simulink model "Tractor_KRAKER_etrailer_v2_2023a_backup050824"  (R2023a)
settings: Solver=VariableStepAuto  StartTime=0.0  StopTime=tmax  FixedStep=dt  RelTol=1e-3  EnableMultiTasking=on
PreLoadFcn:
  | init_vehicle
  | SIMSCAPE_BE_driveline_etrailer_parameters
StartFcn:
  | tic
StopFcn:
  | toc
  | sim_stop_function
  | Etrailer_Simscape_MBM_plotting
undefined symbols (not defined in the file): brake_input, chassis_length, end_val, energyCapacity, etrailer_ON, final_x, final_y, Floor, front_overhang, G, initialSOC, InputSwitch, L_0f, LD, mass_trailer, massload, MaxTrqOut, pose_t0, sp_t, Std_Regen_Trq, steer_input, steer_path, steer_ratio, steer_sens, throttle_input, tire_param_drive, tire_param_steer, tire_param_trailer, tire_width, v_0, Voc, Vx, Vx_input, wheelbase, X, Y, Z
libraries: sm_lib x367, nesl_utility x280, fl_lib x15, sdl_lib x2, robotalgslib x1, simulink_extras x1, batteryecm_lib x1, ee_lib x1, BatteryEstimators x1, CommercialVehicleLibrary2G x1
(part 2 of 12)

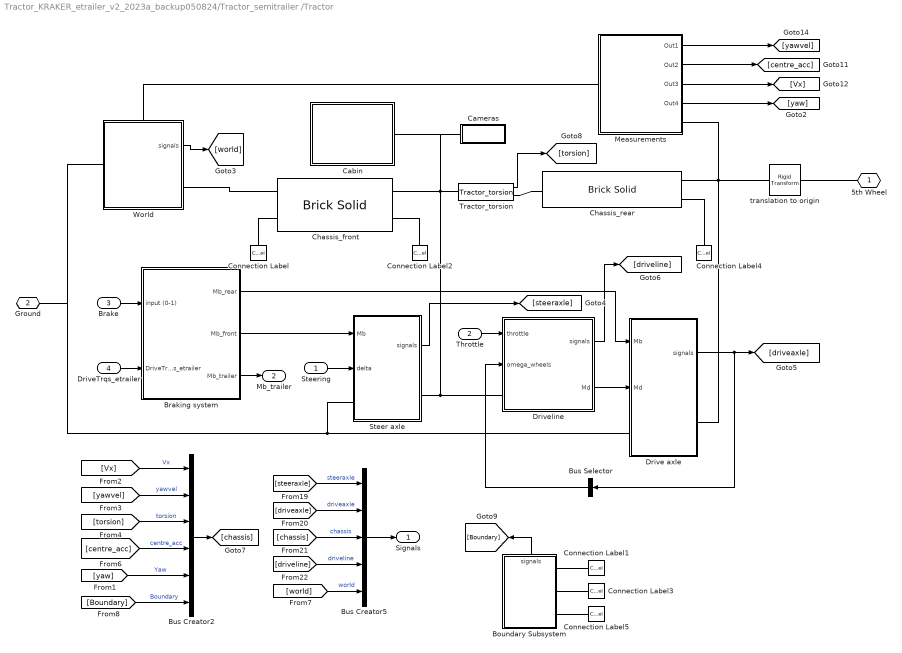
== system Tractor_KRAKER_etrailer_v2_2023a_backup050824/Tractor_semitrailer /Tractor ==
  Steering : Inport
  Throttle : Inport  Port=2
  Brake : Inport  Port=3
  DriveTrqs_etrailer : Inport  Port=4
  Boundary Subsystem : Subsystem
      settings: PortSchema="{\"entries\":[{\"content\":{\"sides\":[{\"content\":{},\"type\":\"ConnectorPlacement.EquallySpacedRectSide\",\"uuid\":\"f1bb1dfb-047a-4b1c-a7c6-7f55b7705282\"},{\"content\":{\"connectorIds\":[\"RConn1\",\"RConn2\",\"RConn3\"],\"side\":\"RIGHT\"},\"type\":\"ConnectorPlacement.EquallySpacedRectSide\",\"uuid\":\"a084a135-f208-49ed-a05d-7dd1e6403e76\"},{\"content\":{\"connectorIds\":[\"Out1\"],\"side\":\"TOP\"},\"type\":\"ConnectorPlacement.EquallySpacedRectSide\",\"uuid\":\"2d0c709c-7e4a-4964-89ae-6ca342da48b8\"},{\"content\":{\"side\":\"BOTTOM\"},\"type\":\"ConnectorPlacement.EquallySpacedRectSide\",\"uuid\":\"a753aab5-92ef-46fc-9973-c1109ebd78e0\"}]},\"type\":\"ConnectorPlacement.EquallySpacedConnector\",\"uuid\":\"ab4af6a2-1912-406b-b131-4cc7a9f5025c\"}],\"packageUris\":[\"http://schema.mathworks.com/mf0/Connector/R2020b\"],\"version\":\"1.0\"}"
      mask Display: disp('Boundary');
  Braking system : Subsystem  AncestorBlock=CommercialVehicleLibrary2G/Components/Braking system
  Bus Creator2 : BusCreator  Inputs=6
  Bus Creator5 : BusCreator  Inputs=5
  Bus Selector : BusSelector  OutputSignals=Omega1,Omega2  OutputAsBus=on
  Cabin : Subsystem  mask(cabin with coil/air suspension){xref=xref+1.10, zref=1.20}
      mask prompts: xref "global X-coordinate cabin tip point [m]"; zref "global Z-coordinate cabin tip point [m]"
      mask Display: disp('Cabin')
  Cameras : Subsystem
  Chassis_front : sm_lib/Body Elements/Brick Solid  GraphicAmbientColor=[0.15 0.15 0.15 1.0]  BasedOnType=Density  BrickDimensions=[l1 w1 h1]  BrickDimensionsUnits=m  CenterOfMass=[0 0 0]  CenterOfMassUnits=m  GraphicDiffuseColor=[0.4 0.4 0.4]  Density=1000  DensityUnits=kg/m^3  DoExposeReferenceFrame=on  GraphicEmissiveColor=[0.0 0.0 0.0 1.0]  ExportEntireGeometry=off  SerializedFrames=<Frames><Frame><Id>Frame1</Id><Value><Name>F1</Name><Origin><Source>ReferenceFrame</Source><FeatureName></FeatureName></Origin><PrimaryAxis><DefinedDirection>+Z</DefinedDirection><Source>ReferenceFrame</Source><SourceDirection>+Z</SourceDirection><FeatureName></FeatureName></PrimaryAxis><SecondaryAxis><DefinedDirection>+X</DefinedDirection><Source>ReferenceFrame</Source><SourceDirection>+X</SourceDirection><FeatureName></FeatureName></SecondaryAxis></Value></Frame><Frame><Id>Frame2</Id><Value><Name>Front</Name><Origin><Source>GeometricFeature</Source><FeatureName>+x surface</FeatureName></Origin><PrimaryAxis><DefinedDirection>+Z</DefinedDirection><Source>ReferenceFrame</Source><SourceDirection>+Z</SourceDirection><FeatureName></FeatureName></PrimaryAxis><SecondaryAxis><DefinedDirection>+X</DefinedDirection><Source>ReferenceFrame</Source><SourceDirection>+X</SourceDirection><FeatureName></FeatureName></SecondaryAxis></Value></Frame><Frame><Id>Frame3</Id><Value><Name>Center</Name><Origin><Source>GeometricFeature</Source><FeatureName>-x surface</FeatureName></Origin><PrimaryAxis><DefinedDirection>+Z</DefinedDirection><Source>ReferenceFrame</Source><SourceDirection>+Z</SourceDirection><FeatureName></FeatureName></PrimaryAxis><SecondaryAxis><DefinedDirection>+X</DefinedDirection><Source>ReferenceFrame</Source><SourceDirection>+X</SourceDirection><FeatureName></FeatureName></SecondaryAxis></Value></Frame></Frames>  MarkerShape=Sphere  MarkerSize=10  GraphicType=FromGeometry  InertiaType=Custom  Mass=front_mass  MassUnits=kg  MomentsOfInertia=[front_Ixx front_Iyy front_Izz]  MomentsOfInertiaUnits=kg*m^2  GraphicOpacity=1  ProductsOfInertia=[0 0 0]  ProductsOfInertiaUnits=kg*m^2  GraphicShininess=75  GraphicSpecularColor=[0.5 0.5 0.5 1.0]  GraphicVisPropType=SimpleVisualProperties
  Chassis_rear : sm_lib/Body Elements/Brick Solid  GraphicAmbientColor=[0.15 0.15 0.15 1.0]  BasedOnType=Density  BrickDimensions=[l2 w2 h2]  BrickDimensionsUnits=m  CenterOfMass=[0 0 0]  CenterOfMassUnits=m  GraphicDiffuseColor=[0.9 0.9 0.9]  Density=1000  DensityUnits=kg/m^3  DoExposeReferenceFrame=on  GraphicEmissiveColor=[0.0 0.0 0.0 1.0]  ExportEntireGeometry=off  SerializedFrames=<Frames><Frame><Id>Frame1</Id><Value><Name>F1</Name><Origin><Source>ReferenceFrame</Source><FeatureName></FeatureName></Origin><PrimaryAxis><DefinedDirection>+Z</DefinedDirection><Source>ReferenceFrame</Source><SourceDirection>+Z</SourceDirection><FeatureName></FeatureName></PrimaryAxis><SecondaryAxis><DefinedDirection>+X</DefinedDirection><Source>ReferenceFrame</Source><SourceDirection>+X</SourceDirection><FeatureName></FeatureName></SecondaryAxis></Value></Frame><Frame><Id>Frame2</Id><Value><Name>Rear</Name><Origin><Source>GeometricFeature</Source><FeatureName>-x surface</FeatureName></Origin><PrimaryAxis><DefinedDirection>+Z</DefinedDirection><Source>ReferenceFrame</Source><SourceDirection>+Z</SourceDirection><FeatureName></FeatureName></PrimaryAxis><SecondaryAxis><DefinedDirection>+X</DefinedDirection><Source>ReferenceFrame</Source><SourceDirection>+X</SourceDirection><FeatureName></FeatureName></SecondaryAxis></Value></Frame></Frames>  MarkerShape=Sphere  MarkerSize=10  GraphicType=FromGeometry  InertiaType=Custom  Mass=rear_mass  MassUnits=kg  MomentsOfInertia=[rear_Ixx rear_Iyy rear_Izz]  MomentsOfInertiaUnits=kg*m^2  GraphicOpacity=0.8  ProductsOfInertia=[0 0 0]  ProductsOfInertiaUnits=kg*m^2  GraphicShininess=75  GraphicSpecularColor=[0.5 0.5 0.5 1.0]  GraphicVisPropType=SimpleVisualProperties
  Connection Label : ConnectionLabel  Label=Center
  Connection Label1 : ConnectionLabel  Label=Center
  Connection Label2 : ConnectionLabel  Label=Front
  Connection Label3 : ConnectionLabel  Label=Front
  Connection Label4 : ConnectionLabel  Label=Rear
  Connection Label5 : ConnectionLabel  Label=Rear
  Drive axle : Subsystem  mask(Driven axle with double tyres){xpos=xref+xrear, tire_param=tire_param_drive, Vx=Vx, Fzstat=Fzstat2}
      mask prompts: xpos "global X-coordinate wheelcentre [m]"; tire_param "tire parameters (structure)"; Vx "initial velocity Vx [m/s]"; Fzstat "initial vertical axle load [N]"
      mask init:
      | Rtyre     = 0.548;
      | Cztyre    = 1.13e+006;
      | tyre_mass = tire_param.INERTIA.MASS;
      | 
      | zpos = Rtyre - 0.25*Fzstat/Cztyre;
      | 
      | tw  =2.15;    % [m], track_width outer tyres
      | ywhl=0.35;   % [m], distance between double tyres
      | yd  =1.00;    % [m], Y-distance bewteen dampers
      | ys  =0.75;    % [m], Y-distance bewteen springs
      | zrc =0.30;   % [m], height of roll centre wrt axle centre 
      | 
      | % damping/stiffness
      | Kspring = 320000;    % [N/m], spring stiffness  (two per axle!)
      | Bdamper =  15000;    % [Ns/m], damper constant  (two per axle!)
      | Kroll   = 500000;    % [Nm/rad] roll stiffness 
      | 
      | % mass/inertia
      | axle_mass =1000;     % [kg] (excl. wheels/tyres!)
      | axle_Ixx  = 380;     % [kgm2]
      | axle_Iyy  =  10;     % [kgm2]
      | axle_Izz  = 380;     % [kgm2]
      |    
      | %rim
      | rim_mass= 50;        % [kg]
      | rim_Ixx =  3;        % [kgm2]
      | rim_Iyy =  5;        % [kgm2] (including rotational inertia brake disk)
      | 
      | %WHeel mass 
      | wheelbody_mass = rim_mass + tire_param.INERTIA.MASS;
      | wheelbody_Ixx  = rim_Ixx  + tire_param.INERTIA.IXX;
      | wheelbody_Iyy  = rim_Iyy  + tire_param.INERTIA.IYY;
      | Imat = [wheelbody_Ixx 0 0; 0 wheelbody_Iyy 0; 0 0 wheelbody_Ixx];
      | sideR=-1;
      | sideL=1;
      | 
      | ld = 0.3;            % loaded spring/damper length
      | ls = ld + 0.5*(Fzstat - 9.81*(axle_mass + 4*tyre_mass + 4*rim_mass))/Kspring;  % spring unloaded length
      settings: LibrarySourceBlock=CommercialVehicleLibrary2G/Assemblies/Drive axle
  Driveline : Subsystem  mask(Engine+gearbox){xref=xref-0.162, zref=0.58, param=DAF XEC + TC-Tronic (355 kW/2100 Nm)}
      mask prompts: xref "global X-coordinate engine ref. point [m]"; zref "global Z-coordinate engine ref. point [m]"; param "parameters"
      mask init:
      | % engine/gearbox: DAF XE355C / ZF 16S221
      | eng_power         = 355000;  % 355 kW
      | max_engine_torque = 2100;    % [Nm]
      | max_revs_rpm      = 1900;    % [rpm]
      | first_gear_ratio  = 16.41;   % [-]
      | final_drive_ratio =  3.07;   % [-]
      |  
      | % engine + gearbox mass (XEC +TC-tronic, DAF 51051/03-042 R. Liebrechts)
      | driveline_mass= 1800;       %[kg]
      | Ixx =  100;       %[kgm2]
      | Iyy =  900;       %[kgm2]
      | Izz =  900;       %[kgm2]
      | yrot=   0;        %[rad] rotation about Y-axis of inertial frame
      | xcg =  -0.25;     %[m], X-coordinate CG wrt rear engine mount ref. point
      | zcg =   0.30;     %[m], Z-coordinate CG wrt rear engine mount ref. point
      |  
      | omega_max=2*pi*max_revs_rpm/60;
      mask TypeOptions param: DAF XEC + TC-Tronic (355 kW/2100 Nm)
  Measurements : Subsystem
  Steer axle : Subsystem  mask(Axle with single tyres and steering system){xpos=xref, tire_param=tire_param_steer, Vx=Vx, Fzstat=Fzstat1}
      mask prompts: xpos "global X-coordinate wheelcentre [m]"; tire_param "tire parameters (structure)"; Vx "initial velocity Vx [m/s]"; Fzstat "initial vertical axle load [N]"
      mask init:
      | Rtyre    = 0.548;
      | Cztyre   = 1.19e+006;
      | tyre_mass= tire_param.INERTIA.MASS;
      | 
      | zpos=Rtyre - 0.5*Fzstat/Cztyre;
      | 
      | steerratio = 20; %[-], ratio steering wheel - front wheels
      |  
      | % dimensions
      | tw =2.0; 	% [m], track_width
      | zrc=0;    	% [m], height of roll centre wrt axle centerline   
      | yd =1.0; 	% [m], Y-distance bewteen dampers 
      | ys =0.85; 	% [m], Y-distance bewteen springs
      | 
      | % stiffness/damping
      | Kspring = 300000;  	% [N/m], spring stiffness (two per axle!)
      | Bdamper =  15000;  	% [Ns/m] damper constant  (two per axle!)
      | Kroll   = 200000;  	% [Nm/rad], roll stiffness 
      |    
      | % mass/inertia   
      | axle_mass = 475;    % [kg] (excl. wheels/tyres!)
      | axle_Ixx  = 200;	% [kgm2]
      | axle_Iyy  = 5;      % [kgm2]
      | axle_Izz  = 200;	% [kgm2]
      |    
      | %rim mass
      | rim_mass= 50; 	% [kg]
      | rim_Ixx =  3; 	% [kgm2]
      | rim_Iyy =  5; 	% [kgm2] (including rotational inertia brake disk)
      | 
      | %WHeel mass 
      | wheelbody_mass = rim_mass + tire_param.INERTIA.MASS;
      | wheelbody_Ixx  = rim_Ixx  + tire_param.INERTIA.IXX;
      | wheelbody_Iyy  = rim_Iyy  + tire_param.INERTIA.IYY;
      | Imat = [wheelbody_Ixx 0 0; 0 wheelbody_Iyy 0; 0 0 wheelbody_Ixx];
      | sideR=-1;
      | sideL=1;
      | 
      | ld = 0.3;       % loaded spring/damper length
      | ls = ld + 0.5*(Fzstat - 9.81*(axle_mass + 2*tyre_mass + 2*rim_mass))/Kspring;  % spring unloaded length
      settings: LibrarySourceBlock=CommercialVehicleLibrary2G/Assemblies/Steer axle
  Tractor_torsion : CommercialVehicleLibrary2G/Components/Tractor_torsion
      mask Display: disp('Torsion');
  World : Subsystem
      settings: LibrarySourceBlock=CommercialVehicleLibrary2G/Utilities/World  PortSchema="{\"entries\":[{\"content\":{\"sides\":[{\"content\":{\"connectorIds\":[\"LConn1\"]},\"type\":\"ConnectorPlacement.EquallySpacedRectSide\",\"uuid\":\"a76c8e8f-6db3-49af-b69e-3287a57a87d6\"},{\"content\":{\"connectorIds\":[\"Out1\",\"RConn1\"],\"side\":\"RIGHT\"},\"type\":\"ConnectorPlacement.EquallySpacedRectSide\",\"uuid\":\"762bfe49-08bc-424a-9ad2-f8d2880b424d\"},{\"content\":{\"connectorIds\":[\"LConn2\"],\"side\":\"TOP\"},\"type\":\"ConnectorPlacement.EquallySpacedRectSide\",\"uuid\":\"ab579a77-7604-4f94-9589-5926789d5e9b\"}]},\"type\":\"ConnectorPlacement.EquallySpacedConnector\",\"uuid\":\"89dbc719-7b2e-4b66-8c99-9a61a858c760\"}],\"packageUris\":[\"http://schema.mathworks.com/mf0/Connector/R2020b\"],\"version\":\"1.0\"}"
  translation to origin : sm_lib/Frames and Transforms/Rigid Transform  TranslationMethod=Cartesian  TranslationStandardOffset=0  TranslationStandardOffsetUnits=m  TranslationStandardAxis=+Z  TranslationCartesianOffset=[-xcg_rear 0 -0.9]  TranslationCartesianOffsetUnits=m  TranslationROffset=0  TranslationROffsetUnits=m  TranslationZOffset=0  TranslationZOffsetUnits=m  TranslationThetaOffset=0  TranslationThetaOffsetUnits=deg  RotationMethod=None  RotationAngleUnits=deg  RotationStandardAxis=+Z  RotationAngle=0.0  RotationArbitraryAxis=[0 0 1]  FollAlignAxisA=+Z  BaseAlignAxisA=+X  FollAlignAxisB=+Y  BaseAlignAxisB=+Y  RotationSequenceAxes=FollowerAxes  RotationSequence=XYX  RotationSequenceAngles=[0 0 0]  RotationSequenceAnglesUnits=deg  RotationMatrix=[1 0 0; 0 1 0; 0 0 1]  Quaternion=[1 0 0 0]
  5th Wheel : PMIOPort  Tag=PMCPort  Side=Right
  Ground : PMIOPort  Port=2  Side=Right
  Signals : Outport
  Mb_trailer : Outport  Port=2
  wires:
  [yawvel] -> Bus Creator2/2  "yawvel"
  Bus Creator2/1 -> [chassis]
  [centre_acc] -> Bus Creator2/4  "centre_acc"
  [torsion] -> Bus Creator2/3  "torsion"
  [Vx] -> Bus Creator2/1  "Vx"
  Tractor_torsion/1 -> [torsion]
  Measurements/3(Out3) -> [Vx]
  Measurements/1(Out1) -> [yawvel]
  Measurements/2(Out2) -> [centre_acc]
  Steer axle/1(signals) -> [steeraxle]
  Drive axle/1(signals) -> Bus Selector/1, [driveaxle]
  Braking system/3(Mb_trailer) -> Mb_trailer/1
  Brake/1 -> Braking system/1(input (0-1))
  Throttle/1 -> Driveline/1(throttle)
  Bus Selector/1 -> Driveline/2(omega_wheels)
  Driveline/2(Md) -> Drive axle/2(Md)
  Steering/1 -> Steer axle/2(delta)
  Driveline/1(signals) -> [driveline]
  [steeraxle] -> Bus Creator5/1  "steeraxle"
  [driveaxle] -> Bus Creator5/2  "driveaxle"
  [chassis] -> Bus Creator5/3  "chassis"
  [driveline] -> Bus Creator5/4  "driveline"
  Bus Creator5/1 -> Signals/1
  Braking system/1(Mb_rear) -> Drive axle/1(Mb)
  Braking system/2(Mb_front) -> Steer axle/1(Mb)
  Measurements/4(Out4) -> [yaw]
  [yaw] -> Bus Creator2/5  "Yaw"
  World/1(signals) -> [world]
  [world] -> Bus Creator5/5  "world"
  Boundary Subsystem/1(signals) -> [Boundary]
  [Boundary] -> Bus Creator2/6  "Boundary"
  DriveTrqs_etrailer/1 -> Braking system/2(DriveTrqs_etrailer)
  connections:
  5th Wheel/RConn1 -- translation to origin/RConn1
  World/RConn1 -- Chassis_front/RConn1
  Chassis_rear/RConn1 -- Tractor_torsion/RConn1
  translation to origin/LConn1 -- Drive axle/RConn1 -- Chassis_rear/LConn1 -- Measurements/RConn1
  World/LConn2 -- Measurements/LConn1
  Steer axle/RConn1 -- Driveline/LConn1 -- Chassis_front/LConn1 -- Cabin/RConn1 -- Cameras/LConn1 -- Tractor_torsion/LConn1
  Drive axle/LConn1 -- Steer axle/LConn1 -- World/LConn1 -- Ground/RConn1
  Chassis_front/RConn2 -- Connection Label/LConn1
  Connection Label1/LConn1 -- Boundary Subsystem/RConn1
  Chassis_front/LConn2 -- Connection Label2/LConn1
  Connection Label3/LConn1 -- Boundary Subsystem/RConn2
  Chassis_rear/LConn2 -- Connection Label4/LConn1
  Connection Label5/LConn1 -- Boundary Subsystem/RConn3

== system Tractor_KRAKER_etrailer_v2_2023a_backup050824/Tractor_semitrailer /Driver/Control ==
  path : Inport
  truck_x : Inport  Port=2
  truck_y : Inport  Port=3
  truck_yaw : Inport  Port=4
  Mux : Mux  Inputs=3
  Pure persuit controller : Subsystem
  Radians to Degrees1 : simulink_extras/Transformations/Radians to Degrees  Commented=on
  Rate Limiter1 : RateLimiter  Commented=on  RisingSlewLimit=0.9  FallingSlewLimit=-0.9  SampleTimeMode=inherited
  Saturation 45 to -45 deg : Saturate  UpperLimit=0.78539816  LowerLimit=-0.78539816
  Simulation end module : Subsystem  Commented=on
  Steering ratio and sens : Gain  Gain=steer_ratio*steer_sens
  delta in rad : Outport
  wires:
  truck_yaw/1 -> Mux/3
  path/1 -> Pure persuit controller/2(Waypoints)
  Pure persuit controller/1(Delta) -> Saturation 45 to -45 deg/1  "delta_C"
  truck_x/1 -> Simulation end module/1(x), Mux/1
  truck_y/1 -> Simulation end module/2(y), Mux/2
  Mux/1 -> Pure persuit controller/1(Pose)
  Steering ratio and sens/1 -> delta in rad/1
  Saturation 45 to -45 deg/1 -> Steering ratio and sens/1

== system Tractor_KRAKER_etrailer_v2_2023a_backup050824/Tractor_semitrailer /Driver/CruiseControl ==
  Vx,ref : Inport
  Vx,actual : Inport  Port=2
  Add : Sum  Inputs=+-
  Add1 : Sum
  Gain : Gain  Gain=5
  Gain1 : Gain  Gain=5
  Integrator : Integrator  InitialCondition=0.0  LimitOutput=on  UpperSaturationLimit=0.1  LowerSaturationLimit=-0.1
  Lookup Table : Lookup  InputValues="[-10  2  10 30]"  Table=[0.04 0.04 1 1]  SaturateOnIntegerOverflow=off
  Product : Product  RndMeth=Zero
  Product1 : Product  RndMeth=Zero
  Scope : Scope  NumInputPorts=2
  To Workspace : ToWorkspace  VariableName=p_velocity_reference  SampleTime=sp_t
  To Workspace1 : ToWorkspace  VariableName=p_velocity_actual  SampleTime=sp_t
  Transfer Fcn : TransferFcn  Denominator=[0.16 1]
  throttle : Outport  VectorParamsAs1DForOutWhenUnconnected=off
  wires:
  Transfer Fcn/1 -> Lookup Table/1
  Lookup Table/1 -> Product/2, Product1/2
  Product1/1 -> Gain1/1
  Product/1 -> Gain/1
  Add/1 -> Product1/1, Product/1
  Add1/1 -> throttle/1
  Gain/1 -> Add1/1
  Integrator/1 -> Add1/2
  Gain1/1 -> Integrator/1
  Vx,ref/1 -> To Workspace/1, Scope/1, Add/1
  Vx,actual/1 -> Transfer Fcn/1, To Workspace1/1, Scope/2, Add/2

== system Tractor_KRAKER_etrailer_v2_2023a_backup050824/Tractor_semitrailer /Driver/Subsystem ==
  Constant : Constant  Value=InputSwitch
  DriveCycle Speed Input : FromWorkspace  VariableName=DrCycles.FTP
  From Workspace : FromWorkspace  VariableName=DrCycles.C505
  From Workspace1 : FromWorkspace  VariableName=DrCycles.UDDS
  From Workspace2 : FromWorkspace  VariableName=DrCycles.HWFET
  From Workspace3 : FromWorkspace  VariableName=DrCycles.US06
  From Workspace4 : FromWorkspace  VariableName=DrCycles.US06City
  From Workspace5 : FromWorkspace  VariableName=DrCycles.US06Hwy
  Multiport Switch : MultiPortSwitch  Inputs=8  SaturateOnIntegerOverflow=off  InputSameDT=off
  Saturation : Saturate  UpperLimit=90  LowerLimit=0
  SineWave DriveCycle Input : Sin  Amplitude=150  Bias=50  Frequency=0.1  SampleTime=0
  mph2mps{,1..6} (7 alike) : Gain  Gain=0.44704
  DriveCycleInput : Outport
  wires:
  SineWave DriveCycle Input/1 -> Saturation/1
  DriveCycle Speed Input/1 -> mph2mps/1
  mph2mps/1 -> Multiport Switch/2
  Constant/1 -> Multiport Switch/1
  Multiport Switch/1 -> DriveCycleInput/1
  mph2mps1/1 -> Multiport Switch/3
  From Workspace/1 -> mph2mps1/1
  mph2mps2/1 -> Multiport Switch/4
  From Workspace1/1 -> mph2mps2/1
  mph2mps3/1 -> Multiport Switch/5
  mph2mps4/1 -> Multiport Switch/6
  mph2mps5/1 -> Multiport Switch/7
  mph2mps6/1 -> Multiport Switch/8
  From Workspace2/1 -> mph2mps3/1
  From Workspace3/1 -> mph2mps4/1
  From Workspace4/1 -> mph2mps5/1
  From Workspace5/1 -> mph2mps6/1
  Saturation/1 -> Multiport Switch/9

== system Tractor_KRAKER_etrailer_v2_2023a_backup050824/Tractor_semitrailer /Kraker etrailer/5th Wheel Joint ==
  note: 2 Joint setup
  note: 1 joint setup
  note: Signals for forces on kingpin
  note: in X-Z-Y
  note: in X-Z-Y
  note: in X-Y-Z
  note: in X-Y-Z
  note: in Z-Y-X
  note: in Z-Y-X
  5th wheel joint : sm_lib/Joints/Revolute Joint  Commented=on  JointMode=Normal  SenseConstraintForce=on  SenseConstraintForceX=off  SenseConstraintForceY=off  SenseConstraintForceZ=off  SenseConstraintTorque=off  SenseConstraintTorqueX=off  SenseConstraintTorqueY=off  SenseConstraintTorqueZ=off  SenseTotalForce=on  SenseTotalForceX=off  SenseTotalForceY=off  SenseTotalForceZ=off  SenseTotalTorque=off  SenseTotalTorqueX=off  SenseTotalTorqueY=off  SenseTotalTorqueZ=off  CompositeWrenchDir=BaseOnFollower  CompositeWrenchFrame=BaseFrame  EquilibriumPosition=0  EquilibriumPositionUnits=deg  SpringStiffness=0  SpringStiffnessUnits=N*m/deg  DampingCoefficient=0  DampingCoefficientUnits=N*m/(deg/s)  TorqueActuationMode=NoTorque  MotionActuationMode=ComputedMotion  SensePosition=off  SenseVelocity=off  SenseAcceleration=off  SenseTorqueForce=off  SenseLowerLimitTorqueForce=off  SenseUpperLimitTorqueForce=off  LowerLimitSpecify=off  LowerLimitBound=-90  LowerLimitBoundUnits=deg  LowerLimitStiffness=1e4  LowerLimitStiffnessUnits=N*m/deg  LowerLimitDamping=10  LowerLimitDampingUnits=N*m/(deg/s)  LowerLimitTransitionRegionWidth=0.1  LowerLimitTransitionRegionWidthUnits=deg  UpperLimitSpecify=off  UpperLimitBound=90  UpperLimitBoundUnits=deg  UpperLimitStiffness=1e4  UpperLimitStiffnessUnits=N*m/deg  UpperLimitDamping=10  UpperLimitDampingUnits=N*m/(deg/s)  UpperLimitTransitionRegionWidth=0.1  UpperLimitTransitionRegionWidthUnits=deg  PositionTargetSpecify=on  PositionTargetPriority=High  PositionTargetValue=-psi_semitrailer  PositionTargetValueUnits=rad  VelocityTargetSpecify=off  VelocityTargetPriority=High  VelocityTargetValue=0  VelocityTargetValueUnits=deg/s
  5th wheel joint - axis : sm_lib/Joints/Revolute Joint  Commented=on  JointMode=Normal  SenseConstraintForce=on  SenseConstraintForceX=off  SenseConstraintForceY=off  SenseConstraintForceZ=off  SenseConstraintTorque=off  SenseConstraintTorqueX=off  SenseConstraintTorqueY=off  SenseConstraintTorqueZ=off  SenseTotalForce=on  SenseTotalForceX=off  SenseTotalForceY=off  SenseTotalForceZ=off  SenseTotalTorque=off  SenseTotalTorqueX=off  SenseTotalTorqueY=off  SenseTotalTorqueZ=off  CompositeWrenchDir=FollowerOnBase  CompositeWrenchFrame=BaseFrame  EquilibriumPosition=0  EquilibriumPositionUnits=deg  SpringStiffness=0  SpringStiffnessUnits=N*m/deg  DampingCoefficient=0  DampingCoefficientUnits=N*m/(deg/s)  TorqueActuationMode=NoTorque  MotionActuationMode=ComputedMotion  SensePosition=off  SenseVelocity=off  SenseAcceleration=off  SenseTorqueForce=off  SenseLowerLimitTorqueForce=off  SenseUpperLimitTorqueForce=off  LowerLimitSpecify=off  LowerLimitBound=-90  LowerLimitBoundUnits=deg  LowerLimitStiffness=1e4  LowerLimitStiffnessUnits=N*m/deg  LowerLimitDamping=10  LowerLimitDampingUnits=N*m/(deg/s)  LowerLimitTransitionRegionWidth=0.1  LowerLimitTransitionRegionWidthUnits=deg  UpperLimitSpecify=off  UpperLimitBound=90  UpperLimitBoundUnits=deg  UpperLimitStiffness=1e4  UpperLimitStiffnessUnits=N*m/deg  UpperLimitDamping=10  UpperLimitDampingUnits=N*m/(deg/s)  UpperLimitTransitionRegionWidth=0.1  UpperLimitTransitionRegionWidthUnits=deg  PositionTargetSpecify=off  PositionTargetPriority=High  PositionTargetValue=0  PositionTargetValueUnits=deg  VelocityTargetSpecify=off  VelocityTargetPriority=High  VelocityTargetValue=0  VelocityTargetValueUnits=deg/s
  Align : sm_lib/Frames and Transforms/Rigid Transform  TranslationMethod=None  TranslationStandardOffset=0  TranslationStandardOffsetUnits=m  TranslationStandardAxis=+Z  TranslationCartesianOffset=[0 0 0]  TranslationCartesianOffsetUnits=m  TranslationROffset=0  TranslationROffsetUnits=m  TranslationZOffset=0  TranslationZOffsetUnits=m  TranslationThetaOffset=0  TranslationThetaOffsetUnits=deg  RotationMethod=AlignedAxes  RotationAngleUnits=deg  RotationStandardAxis=+Z  RotationAngle=0.0  RotationArbitraryAxis=[0 0 1]  FollAlignAxisA=+X  BaseAlignAxisA=+Z  FollAlignAxisB=+Y  BaseAlignAxisB=+Y  RotationSequenceAxes=FollowerAxes  RotationSequence=XYX  RotationSequenceAngles=[0 0 0]  RotationSequenceAnglesUnits=deg  RotationMatrix=[1 0 0; 0 1 0; 0 0 1]  Quaternion=[1 0 0 0]
  Align_5th wheel : sm_lib/Frames and Transforms/Rigid Transform  Commented=on  TranslationMethod=None  TranslationStandardOffset=0  TranslationStandardOffsetUnits=m  TranslationStandardAxis=+Z  TranslationCartesianOffset=[0 0 0]  TranslationCartesianOffsetUnits=m  TranslationROffset=0  TranslationROffsetUnits=m  TranslationZOffset=0  TranslationZOffsetUnits=m  TranslationThetaOffset=0  TranslationThetaOffsetUnits=deg  RotationMethod=AlignedAxes  RotationAngleUnits=deg  RotationStandardAxis=+Z  RotationAngle=0.0  RotationArbitraryAxis=[0 0 1]  FollAlignAxisA=+Z  BaseAlignAxisA=+Y  FollAlignAxisB=+X  BaseAlignAxisB=+X  RotationSequenceAxes=FollowerAxes  RotationSequence=XYX  RotationSequenceAngles=[0 0 0]  RotationSequenceAnglesUnits=deg  RotationMatrix=[1 0 0; 0 1 0; 0 0 1]  Quaternion=[1 0 0 0]
  Bus Creator : BusCreator  Inputs=3
  Bus Creator1 : BusCreator  Inputs=5
  Goto1 : Goto  Commented=on  GotoTag=Ft_Joint1
  Goto2 : Goto  Commented=on  GotoTag=Fc_Joint1
  Goto3 : Goto  Commented=on  GotoTag=Ft_Joint2
  Goto4 : Goto  Commented=on  GotoTag=Fc_Joint2
  PS-Simulink Converter : nesl_utility/PS-Simulink Converter  PhysicalDomain=network_engine_domain  SubClassName=ps_output  LeftPortType=input  RightPortType=output  PseudoPeriodic=off  Frequencies=[]  VectorFormat=1-D array  Unit=inherit  AffineConversion=off
  PS-Simulink Converter1 : nesl_utility/PS-Simulink Converter  PhysicalDomain=network_engine_domain  SubClassName=ps_output  LeftPortType=input  RightPortType=output  PseudoPeriodic=off  Frequencies=[]  VectorFormat=1-D array  Unit=inherit  AffineConversion=off
  PS-Simulink Converter10 : nesl_utility/PS-Simulink Converter  PhysicalDomain=network_engine_domain  SubClassName=ps_output  LeftPortType=input  RightPortType=output  PseudoPeriodic=off  Frequencies=[]  VectorFormat=1-D array  Unit=deg  AffineConversion=off
  PS-Simulink Converter2 : nesl_utility/PS-Simulink Converter  PhysicalDomain=network_engine_domain  SubClassName=ps_output  LeftPortType=input  RightPortType=output  PseudoPeriodic=off  Frequencies=[]  VectorFormat=1-D array  Unit=inherit  AffineConversion=off
  PS-Simulink Converter{3..6} (4 alike) : nesl_utility/PS-Simulink Converter  Commented=on  PhysicalDomain=network_engine_domain  SubClassName=ps_output  LeftPortType=input  RightPortType=output  PseudoPeriodic=off  Frequencies=[]  VectorFormat=1-D array  Unit=N  AffineConversion=off
  PS-Simulink Converter8 : nesl_utility/PS-Simulink Converter  PhysicalDomain=network_engine_domain  SubClassName=ps_output  LeftPortType=input  RightPortType=output  PseudoPeriodic=off  Frequencies=[]  VectorFormat=1-D array  Unit=N  AffineConversion=off
  PS-Simulink Converter9 : nesl_utility/PS-Simulink Converter  PhysicalDomain=network_engine_domain  SubClassName=ps_output  LeftPortType=input  RightPortType=output  PseudoPeriodic=off  Frequencies=[]  VectorFormat=1-D array  Unit=N  AffineConversion=off
  Realign : sm_lib/Frames and Transforms/Rigid Transform  TranslationMethod=None  TranslationStandardOffset=0  TranslationStandardOffsetUnits=m  TranslationStandardAxis=+Z  TranslationCartesianOffset=[0 0 0]  TranslationCartesianOffsetUnits=m  TranslationROffset=0  TranslationROffsetUnits=m  TranslationZOffset=0  TranslationZOffsetUnits=m  TranslationThetaOffset=0  TranslationThetaOffsetUnits=deg  RotationMethod=AlignedAxes  RotationAngleUnits=deg  RotationStandardAxis=+Z  RotationAngle=0.0  RotationArbitraryAxis=[0 0 1]  FollAlignAxisA=+Z  BaseAlignAxisA=+X  FollAlignAxisB=+Y  BaseAlignAxisB=+Y  RotationSequenceAxes=FollowerAxes  RotationSequence=XYX  RotationSequenceAngles=[0 0 0]  RotationSequenceAnglesUnits=deg  RotationMatrix=[1 0 0; 0 1 0; 0 0 1]  Quaternion=[1 0 0 0]
  Realign_5th wheel : sm_lib/Frames and Transforms/Rigid Transform  Commented=on  TranslationMethod=None  TranslationStandardOffset=0  TranslationStandardOffsetUnits=m  TranslationStandardAxis=+Z  TranslationCartesianOffset=[0 0 0]  TranslationCartesianOffsetUnits=m  TranslationROffset=0  TranslationROffsetUnits=m  TranslationZOffset=0  TranslationZOffsetUnits=m  TranslationThetaOffset=0  TranslationThetaOffsetUnits=deg  RotationMethod=AlignedAxes  RotationAngleUnits=deg  RotationStandardAxis=+Z  RotationAngle=0.0  RotationArbitraryAxis=[0 0 1]  FollAlignAxisA=+Y  BaseAlignAxisA=+Z  FollAlignAxisB=+X  BaseAlignAxisB=+X  RotationSequenceAxes=FollowerAxes  RotationSequence=XYX  RotationSequenceAngles=[0 0 0]  RotationSequenceAnglesUnits=deg  RotationMatrix=[1 0 0; 0 1 0; 0 0 1]  Quaternion=[1 0 0 0]
  Scope : Scope
  Transform Sensor : sm_lib/Frames and Transforms/Transform Sensor  MeasurementFrame=World  RotationSequence=XYX  SenseAngle=off  SenseAxis=off  SenseQ=off  SenseR=off  SenseRotationSequence=off  SenseOmegaX=off  SenseOmegaY=off  SenseOmegaZ=off  SenseQDot=off  SenseRDot=off  SenseRotationSequenceDot=off  SenseAlphaX=off  SenseAlphaY=off  SenseAlphaZ=off  SenseQDDot=off  SenseRDDot=off  SenseX=on  SenseY=on  SenseZ=on  SenseRad=off  SenseAzim=off  SenseDist=off  SenseInc=off  SenseXDot=off  SenseYDot=off  SenseZDot=off  SenseRadDot=off  SenseAzimDot=off  SenseDistDot=off  SenseIncDot=off  SenseXDDot=off  SenseYDDot=off  SenseZDDot=off  SenseRadDDot=off  SenseAzimDDot=off  SenseDistDDot=off  SenseIncDDot=off
  Universal Joint : sm_lib/Joints/Universal Joint  JointMode=Normal  SenseConstraintForce=on  SenseConstraintForceX=off  SenseConstraintForceY=off  SenseConstraintForceZ=off  SenseConstraintTorque=off  SenseConstraintTorqueX=off  SenseConstraintTorqueY=off  SenseConstraintTorqueZ=off  SenseTotalForce=on  SenseTotalForceX=off  SenseTotalForceY=off  SenseTotalForceZ=off  SenseTotalTorque=off  SenseTotalTorqueX=off  SenseTotalTorqueY=off  SenseTotalTorqueZ=off  CompositeWrenchDir=FollowerOnBase  CompositeWrenchFrame=FollowerFrame  RxEquilibriumPosition=0  RxEquilibriumPositionUnits=deg  RxSpringStiffness=0  RxSpringStiffnessUnits=N*m/deg  RxDampingCoefficient=0  RxDampingCoefficientUnits=N*m/(deg/s)  RxTorqueActuationMode=NoTorque  RxMotionActuationMode=ComputedMotion  RxSensePosition=off  RxSenseVelocity=off  RxSenseAcceleration=off  RxSenseTorqueForce=off  RxSenseLowerLimitTorqueForce=off  RxSenseUpperLimitTorqueForce=off  RxLowerLimitSpecify=off  RxLowerLimitBound=-90  RxLowerLimitBoundUnits=deg  RxLowerLimitStiffness=1e4  RxLowerLimitStiffnessUnits=N*m/deg  RxLowerLimitDamping=10  RxLowerLimitDampingUnits=N*m/(deg/s)  RxLowerLimitTransitionRegionWidth=0.1  RxLowerLimitTransitionRegionWidthUnits=deg  RxUpperLimitSpecify=off  RxUpperLimitBound=90  RxUpperLimitBoundUnits=deg  RxUpperLimitStiffness=1e4  RxUpperLimitStiffnessUnits=N*m/deg  RxUpperLimitDamping=10  RxUpperLimitDampingUnits=N*m/(deg/s)  RxUpperLimitTransitionRegionWidth=0.1  RxUpperLimitTransitionRegionWidthUnits=deg  RxPositionTargetSpecify=off  RxPositionTargetPriority=High  RxPositionTargetValue=0  RxPositionTargetValueUnits=deg  RxVelocityTargetSpecify=off  RxVelocityTargetPriority=High  RxVelocityTargetValue=0  RxVelocityTargetValueUnits=deg/s  RyEquilibriumPosition=0  RyEquilibriumPositionUnits=deg  RySpringStiffness=0  RySpringStiffnessUnits=N*m/deg  RyDampingCoefficient=0  RyDampingCoefficientUnits=N*m/(deg/s)  RyTorqueActuationMode=NoTorque  RyMotionActuationMode=ComputedMotion  RySensePosition=on  RySenseVelocity=off  RySenseAcceleration=off  RySenseTorqueForce=off  RySenseLowerLimitTorqueForce=off  RySenseUpperLimitTorqueForce=off  RyLowerLimitSpecify=off  RyLowerLimitBound=-90  RyLowerLimitBoundUnits=deg  RyLowerLimitStiffness=1e4  RyLowerLimitStiffnessUnits=N*m/deg  RyLowerLimitDamping=10  RyLowerLimitDampingUnits=N*m/(deg/s)  RyLowerLimitTransitionRegionWidth=0.1  RyLowerLimitTransitionRegionWidthUnits=deg  RyUpperLimitSpecify=off  RyUpperLimitBound=90  RyUpperLimitBoundUnits=deg  RyUpperLimitStiffness=1e4  RyUpperLimitStiffnessUnits=N*m/deg  RyUpperLimitDamping=10  RyUpperLimitDampingUnits=N*m/(deg/s)  RyUpperLimitTransitionRegionWidth=0.1  RyUpperLimitTransitionRegionWidthUnits=deg  RyPositionTargetSpecify=off  RyPositionTargetPriority=High  RyPositionTargetValue=0  RyPositionTargetValueUnits=deg  RyVelocityTargetSpecify=off  RyVelocityTargetPriority=High  RyVelocityTargetValue=0  RyVelocityTargetValueUnits=deg/s
  World Frame : sm_lib/Frames and Transforms/World Frame
  pos_5th Wheel : sm_lib/Frames and Transforms/Rigid Transform  TranslationMethod=Cartesian  TranslationStandardOffset=0  TranslationStandardOffsetUnits=m  TranslationStandardAxis=+Z  TranslationCartesianOffset=[xref 0 1.15]  TranslationCartesianOffsetUnits=m  TranslationROffset=0  TranslationROffsetUnits=m  TranslationZOffset=0  TranslationZOffsetUnits=m  TranslationThetaOffset=0  TranslationThetaOffsetUnits=deg  RotationMethod=None  RotationAngleUnits=deg  RotationStandardAxis=+Z  RotationAngle=0.0  RotationArbitraryAxis=[0 0 1]  FollAlignAxisA=+X  BaseAlignAxisA=+Y  FollAlignAxisB=+Y  BaseAlignAxisB=+Z  RotationSequenceAxes=FollowerAxes  RotationSequence=XYX  RotationSequenceAngles=[0 0 0]  RotationSequenceAnglesUnits=deg  RotationMatrix=[1 0 0; 0 1 0; 0 0 1]  Quaternion=[1 0 0 0]
  pos_trailer_front : sm_lib/Frames and Transforms/Rigid Transform  TranslationMethod=Cartesian  TranslationStandardOffset=1.8  TranslationStandardOffsetUnits=m  TranslationStandardAxis=-X  TranslationCartesianOffset=[-xref+xcg1 0 0.05]  TranslationCartesianOffsetUnits=m  TranslationROffset=0  TranslationROffsetUnits=m  TranslationZOffset=0  TranslationZOffsetUnits=m  TranslationThetaOffset=0  TranslationThetaOffsetUnits=deg  RotationMethod=None  RotationAngleUnits=deg  RotationStandardAxis=+Z  RotationAngle=0.0  RotationArbitraryAxis=[0 0 1]  FollAlignAxisA=+X  BaseAlignAxisA=+Y  FollAlignAxisB=+Y  BaseAlignAxisB=+Z  RotationSequenceAxes=FollowerAxes  RotationSequence=XYX  RotationSequenceAngles=[0 0 0]  RotationSequenceAnglesUnits=deg  RotationMatrix=[1 0 0; 0 1 0; 0 0 1]  Quaternion=[1 0 0 0]
  Chassis : PMIOPort  Side=Left
  Trailer : PMIOPort  Port=2  Side=Right
  signals : Outport
  wires:
  Bus Creator/1 -> [pos]
  PS-Simulink Converter1/1 -> Bus Creator/2  "Y"
  PS-Simulink Converter2/1 -> Bus Creator/3  "Z"
  PS-Simulink Converter/1 -> Bus Creator/1  "X"
  [Fc_Joint1] -> Bus Creator1/3  "fc_joint1"
  Bus Creator1/1 -> signals/1
  [Ft_Joint1] -> Bus Creator1/2  "ft_joint1"
  [pos] -> Bus Creator1/1  "pos"
  [Fc_Joint2] -> Bus Creator1/5  "fc_joint2"
  [Ft_Joint2] -> Bus Creator1/4  "ft_joint2"
  PS-Simulink Converter3/1 -> Goto1/1  "Force"
  PS-Simulink Converter5/1 -> Goto2/1  "Force"
  PS-Simulink Converter4/1 -> Goto3/1  "Force"
  PS-Simulink Converter6/1 -> Goto4/1  "Force"
  PS-Simulink Converter9/1 -> [Ft_Joint1]  "Force"
  PS-Simulink Converter8/1 -> [Fc_Joint1]  "Force"
  PS-Simulink Converter10/1 -> Scope/1  "Angle"
  connections:
  pos_5th Wheel/LConn1 -- Chassis/RConn1
  Transform Sensor/RConn1 -- Align/LConn1 -- pos_5th Wheel/RConn1
  pos_trailer_front/RConn1 -- Trailer/RConn1
  5th wheel joint/LConn1 -- Realign_5th wheel/RConn1
  5th wheel joint - axis/RConn1 -- Realign_5th wheel/LConn1
  Align_5th wheel/RConn1 -- 5th wheel joint - axis/LConn1
  World Frame/RConn1 -- Transform Sensor/LConn1
  PS-Simulink Converter2/LConn1 -- Transform Sensor/RConn4
  PS-Simulink Converter1/LConn1 -- Transform Sensor/RConn3
  PS-Simulink Converter/LConn1 -- Transform Sensor/RConn2
  PS-Simulink Converter3/LConn1 -- 5th wheel joint - axis/RConn3
  PS-Simulink Converter5/LConn1 -- 5th wheel joint - axis/RConn2
  PS-Simulink Converter4/LConn1 -- 5th wheel joint/RConn3
  PS-Simulink Converter6/LConn1 -- 5th wheel joint/RConn2
  Universal Joint/RConn1 -- Realign/LConn1
  Universal Joint/LConn1 -- Align/RConn1
  PS-Simulink Converter8/LConn1 -- Universal Joint/RConn3
  PS-Simulink Converter10/LConn1 -- Universal Joint/RConn2
  pos_trailer_front/LConn1 -- Realign/RConn1
  PS-Simulink Converter9/LConn1 -- Universal Joint/RConn4

== system Tractor_KRAKER_etrailer_v2_2023a_backup050824/Tractor_semitrailer /Kraker etrailer/Cameras ==
  Trailer Camera Position : sm_lib/Frames and Transforms/Rigid Transform  TranslationMethod=Cartesian  TranslationStandardOffset=0  TranslationStandardOffsetUnits=m  TranslationStandardAxis=+Z  TranslationCartesianOffset=[-20 0 8]  TranslationCartesianOffsetUnits=m  TranslationROffset=0  TranslationROffsetUnits=m  TranslationZOffset=0  TranslationZOffsetUnits=m  TranslationThetaOffset=0  TranslationThetaOffsetUnits=deg  RotationMethod=None  RotationAngleUnits=deg  RotationStandardAxis=+Z  RotationAngle=0.0  RotationArbitraryAxis=[0 0 1]  FollAlignAxisA=+X  BaseAlignAxisA=+Y  FollAlignAxisB=+Y  BaseAlignAxisB=+Z  RotationSequenceAxes=FollowerAxes  RotationSequence=XYX  RotationSequenceAngles=[0 0 0]  RotationSequenceAnglesUnits=deg  RotationMatrix=[1 0 0; 0 1 0; 0 0 1]  Quaternion=[1 0 0 0]
  Trailer Camera Sphere : sm_lib/Body Elements/Spherical Solid  GraphicAmbientColor=[0.15 0.15 0.15 1.0]  BasedOnType=Density  CenterOfMass=[0 0 0]  CenterOfMassUnits=m  GraphicDiffuseColor=[0.5 0.5 0.5]  Density=1000  DensityUnits=kg/m^3  DoExposeReferenceFrame=on  GraphicEmissiveColor=[0.0 0.0 0.0 1.0]  ExportEntireGeometry=off  SerializedExposedGeometries=<ExposedGeometries/>  SerializedFrames=<Frames/>  MarkerShape=Sphere  MarkerSize=10  GraphicType=FromGeometry  InertiaType=PointMass  Mass=1e-10  MassUnits=kg  MomentsOfInertia=[1 1 1]  MomentsOfInertiaUnits=kg*m^2  GraphicOpacity=0  ProductsOfInertia=[0 0 0]  ProductsOfInertiaUnits=kg*m^2  GraphicShininess=75  GraphicSpecularColor=[0.5 0.5 0.5 1.0]  SphereRadius=1e-10  SphereRadiusUnits=m  GraphicVisPropType=SimpleVisualProperties
  " " : PMIOPort  Side=Right
  connections:
  Trailer Camera Position/LConn1 -- " "/RConn1
  Trailer Camera Sphere/RConn1 -- Trailer Camera Position/RConn1

== system Tractor_KRAKER_etrailer_v2_2023a_backup050824/Tractor_semitrailer /Kraker etrailer/Electric Powertrain ==
  MotCmdTrq : Inport
  Add : Sum  Inputs=+-
  Battery model : batteryecm_lib/Battery  Vnom=Voc V  prm_dir=simscape.enum.battery.prm_dir.disabled  R1_dis=2 Ohm  R1_ch=2 Ohm  R1=Rin Ohm  prm_AH=simscape.enum.battery.prm_AH.finite  AH=energyCapacity A*hr  V1=Voc*(11.5/12) V  AH1=energyCapacity*(11.5/12) A*hr  prm_R2=simscape.enum.battery.prm_R2.disabled  R2=2000 Ohm  Tmeas=298.15 K  charge_measurement_port=simscape.enum.battery.enable.no  prm_dyn=simscape.enum.battery.prm_dyn.off  Rp1=0.005 Ohm  tau1=30 s  Rp2=0.005 Ohm  tau2=30 s  Rp3=0.005 Ohm  tau3=30 s  Rp4=0.005 Ohm  tau4=30 s  Rp5=0.005 Ohm  tau5=30 s  prm_fade=simscape.enum.battery.prm_fade.disabled  N_fade=100  AH_fade=45 A*hr  R1_fade=2.02 Ohm  R1_ch_fade=2.02 Ohm  V1_fade=10.35 V  prm_age=simscape.enum.battery.prm_age.disabled  prm_age_OCV=simscape.enum.battery.prm_age_OCV.OCV  OCV_age=0.9  SOC_age=60  Tmeas_age=298.15 K  delta_time_age_vec=[0] d  temperature_age_vec=[273] K  OCV_scaling_age=2.2134e6  OCV_offset_age=1.632e6  temp_exp_age=0.515833569 V  t_exp_age=0.75  Vnom_T2=675 V  R1_T2=Rin Ohm  R1_T2_dis=2.2 Ohm  R1_T2_ch=2.2 Ohm  V1_T2=660 V  R2_T2=2200 Ohm  Rp1_T2=0.005 Ohm  tau1_T2=30 s  Rp2_T2=0.005 Ohm  tau2_T2=30 s  Rp3_T2=0.005 Ohm  tau3_T2=30 s  Rp4_T2=0.005 Ohm  tau4_T2=30 s  Rp5_T2=0.005 Ohm  tau5_T2=30 s  Tmeas2=273.15 K  thermal_port=simscape.enum.thermaleffects.model  thermal_mass=30000 J/K  i_specify=off  i_priority=None  i=0 A  i_nominal_specify=off  i_nominal_unit=A  i_nominal_value=1  v_specify=off  v_priority=None  v=0 V  v_nominal_specify=off  v_nominal_unit=V  v_nominal_value=1  charge_specify=on  charge_priority=High  charge=energyCapacity*initialSOC A*hr  charge_nominal_specify=off  charge_nominal_unit=A*hr  charge_nominal_value=1  num_cycles_specify=off  num_cycles_priority=High  num_cycles=0  num_cycles_nominal_specify=off  num_cycles_nominal_unit=1  num_cycles_nominal_value=1  temperature_specify=off  temperature_priority=High  temperature=298.15 K  temperature_nominal_specify=off  temperature_nominal_unit=K  temperature_nominal_value=1
      settings: InternalSimscapePortConfiguration="{\"Bottom\":[],\"Left\":[{\"id\":\"p\",\"label\":\"+\",\"type\":\"foundation.electrical.electrical\"}],\"Right\":[{\"id\":\"n\",\"label\":\"-\",\"type\":\"foundation.electrical.electrical\"},{\"id\":\"H\",\"label\":\"H\",\"type\":\"foundation.thermal.thermal\"}],\"Top\":[]}"
  Constant : Constant  Value=273
  Electrical Reference : fl_lib/Electrical/Electrical Elements/Electrical Reference
  Electrical Reference1 : fl_lib/Electrical/Electrical Elements/Electrical Reference
  Mechanical Rotational Reference : fl_lib/Mechanical/Rotational Elements/Mechanical Rotational Reference
  Motor Reducer : sdl_lib/Gears/Simple Gear  ratio=1  rotation_direction=3-2*(1)  friction_model=sdl.enum.gear_efficiencies_load.off  T_noload=0.1 N*m  T_nom=5 N*m  efficiency_nom=0.8  efficiency=0.8  temperature_TLU=[280, 300, 320] K  load_TLU=[1, 5, 10] N*m  efficiency_TLU=[.95, .9, .85]  efficiency_TLU2=[.85, .8, .75; .95, .9, .85; .85, .8, .7]  w_thr=0.01 rad/s  pwr_thr=0.001 W  enable_backlash=false  hardstop_model=simscape.enum.hardstop.smooth  backlash_distance=1e-3 mm  r_base=0.1 m  transition=1e-4 mm  backlash_stiffness=1e7 N/m  backlash_damping=1e6 N*s/m  coeff_rest=0  v_tol=0.001 m/s  f_tol=0 N  mu_visc=[0, 0] N*m/(rad/s)  enable_faults=simscape.enum.onoff.off  efficiency_fault=0.05  external_fault=simscape.enum.onoff.off  temporal_fault=simscape.enum.onoff.off  fault_time=5 s  fault_angles=pi / 12 rad  report_fault=(1)-1  thermal_mass=50 J/K  temperature_specify=off  temperature_priority=High  temperature=300 K  temperature_nominal_specify=off  temperature_nominal_unit=K  temperature_nominal_value=1  x_backlash_specify=off  x_backlash_priority=None  x_backlash=0 mm  x_backlash_nominal_specify=off  x_backlash_nominal_unit=mm  x_backlash_nominal_value=1  f_hardstop_specify=off  f_hardstop_priority=None  f_hardstop=0 N  f_hardstop_nominal_specify=off  f_hardstop_nominal_unit=N  f_hardstop_nominal_value=1  v_backlash_specify=off  v_backlash_priority=None  v_backlash=0 m/s  v_backlash_nominal_specify=off  v_backlash_nominal_unit=m/s  v_backlash_nominal_value=1
  Motor & Drive (System Level) : ee_lib/Electromechanical/Motor & Drive (System Level)  torque_speed_param=ee.enum.electromech.envelope.torque_power  overtorque_param=ee.enum.electromech.overtorque.no  T_t=[.09, .08, .07, 0] N*m  T_t_intermittent=[.36, .32, .28, 0] N*m  T_t_2D=[.09, .09, .09; .08, .08, .08; .07, .07, .07; 0, 0, 0] N*m  T_t_intermittent_2D=[.36, .36, .36; .32, .32, .32; .28, .28, .28; 0, 0, 0] N*m  w_t=[0, 3750, 7500, 8000] rpm  vdc_t=[6, 12, 24] V  torque_max=MaxTrqOut N*m  power_max=MaxPowerOut W  torque_max_intermittent=0.4 N*m  power_max_intermittent=120 W  time_overtorque=30 s  time_recover=60 s  Tc=0.2 s  losses_param=1  eff=100  w_eff=3750 rpm  T_eff=0.08 N*m  Piron=0 W  Pbase=0 W  w_eff_vec=motorDrive.simplePmsmDrv_spdVec_rpm rpm  T_eff_vec=motorDrive.simplePmsmDrv_trqVec_Nm N*m  v_eff_vec=[100, 250, 400] V  losses_mat=motorDrive.simplePmsmDrv_LossTbl_W W  efficiency_mat=[95, 95, 95, 95; 95, 95, 95, 95; 95, 95, 95, 95; 95, 95, 95, 95; 95, 95, 95, 95]  losses_mat_3D=ones(5, 4, 3) W  efficiency_mat_3D=95 * ones(5, 4, 3)  Res=0 Ohm  enable_fault=simscape.enum.onoff.off  fault_condition=1  fault_threshold=0.5  J=1.3100e-04 kg*m^2  lam=1e-05 N*m/(rad/s)  speed0=0 rpm  faulted_specify=off  faulted_priority=None  faulted=0  faulted_nominal_specify=off  faulted_nominal_unit=1  faulted_nominal_value=1  torqueLimitContinuous_specify=off  torqueLimitContinuous_priority=None  torqueLimitContinuous=0 N*m  torqueLimitContinuous_nominal_specify=off  torqueLimitContinuous_nominal_unit=N*m  torqueLimitContinuous_nominal_value=1  alpha=3.93e-3 1/K  Tmeas=25 degC  Tmeas2=125 degC  losses_mat_T2=motorDrive.simplePmsmDrv_LossTbl_W W  efficiency_mat_T2=[95, 95, 95, 95; 95, 95, 95, 95; 95, 95, 95, 95; 95, 95, 95, 95; 95, 95, 95, 95]  losses_mat_3D_T2=ones(5, 4, 3) W  efficiency_mat_3D_T2=95 * ones(5, 4, 3)  thermal_mass=10 J/K  initial_temperature=100 degC
      settings: LogSimulationData=on  InternalSimscapePortConfiguration="{\"Bottom\":[],\"Left\":[{\"id\":\"Vp\",\"label\":\"+\",\"type\":\"foundation.electrical.electrical\"},{\"id\":\"Tr\",\"label\":\"Tr\",\"type\":\"input\"},{\"id\":\"R\",\"label\":\"R\",\"type\":\"foundation.mechanical.rotational.rotational\"}],\"Right\":[{\"id\":\"Vm\",\"label\":\"-\",\"type\":\"foundation.electrical.electrical\"},{\"id\":\"Omega\",\"label\":\"w\",\"type\":\"output\"},{\"id\":\"H\",\"label\":\"H\",\"type\":\"foundation.thermal.thermal\"},{\"id\":\"C\",\"label\":\"C\",\"type\":\"foundation.mechanical.rotational.rotational\"}],\"Top\":[]}"
  PS Terminator : fl_lib/Physical Signals/Sinks/PS Terminator
  PS-Simulink Converter1 : nesl_utility/PS-Simulink Converter  PhysicalDomain=network_engine_domain  SubClassName=ps_output  LeftPortType=input  RightPortType=output  PseudoPeriodic=off  Frequencies=[]  VectorFormat=1-D array  Unit=1  AffineConversion=off
  PS-Simulink Converter2 : nesl_utility/PS-Simulink Converter  PhysicalDomain=network_engine_domain  SubClassName=ps_output  LeftPortType=input  RightPortType=output  PseudoPeriodic=off  Frequencies=[]  VectorFormat=1-D array  Unit=V  AffineConversion=off
  Perfect Insulator : fl_lib/Thermal/Thermal Elements/Perfect Insulator  T_specify=off  T_priority=None  T=293.15 K  T_nominal_specify=off  T_nominal_unit=K  T_nominal_value=1
  SOC calculation : Subsystem
  Simulink-PS Converter1 : nesl_utility/Simulink-PS Converter  PhysicalDomain=network_engine_domain  SubClassName=ps_input  LeftPortType=input  RightPortType=output  PseudoPeriodic=off  Frequencies=[]  NoiseDistribution=none  NoiseParameters=[]  Unit=N*m  AffineConversion=off  FilteringAndDerivatives=provide  SimscapeFilterOrder=1  InputFilterTimeConstant=0.001  UdotUserProvided=0
  Speed Sensor : Subsystem
      mask Display: disp('w')
  Temperature Sensor : fl_lib/Thermal/Thermal Sensors/Temperature Sensor  temperature_measure=foundation.enum.MeasurementReference.absolute
      settings: InternalSimscapePortConfiguration="{\"Bottom\":[],\"Left\":[{\"id\":\"A\",\"label\":\"A\",\"type\":\"foundation.thermal.thermal\"}],\"Right\":[{\"id\":\"T\",\"label\":\"T\",\"type\":\"output\"}],\"Top\":[]}"
  To Workspace : ToWorkspace  VariableName=p_battery_SOCcoulomb  SampleTime=sp_t
  To Workspace1 : ToWorkspace  VariableName=p_battery_SOCcalc  SampleTime=sp_t
  To Workspace2 : ToWorkspace  VariableName=p_battery_current  SampleTime=sp_t
  To Workspace3 : ToWorkspace  VariableName=p_battery_temperature  SampleTime=sp_t
  To Workspace4 : ToWorkspace  VariableName=p_battery_Voc  SampleTime=sp_t
  To Workspace5 : ToWorkspace  VariableName=p_Emotor_speed  SampleTime=sp_t
  Voltage Sensor : fl_lib/Electrical/Electrical Sensors/Voltage Sensor
  MotorShaftOut : PMIOPort  Side=Right
  SOC : Outport
  wires:
  Speed Sensor/1(w) -> To Workspace5/1
  MotCmdTrq/1 -> Simulink-PS Converter1/1
  SOC calculation/2(Current) -> To Workspace2/1
  SOC calculation/1(SOC_Coulomb) -> To Workspace/1
  PS-Simulink Converter1/1 -> Add/1
  Add/1 -> To Workspace3/1
  Constant/1 -> Add/2
  SOC calculation/3(SOC_calc) -> SOC/1, To Workspace1/1
  PS-Simulink Converter2/1 -> To Workspace4/1, SOC calculation/1(Voc)
  connections:
  Electrical Reference/LConn1 -- Motor & Drive (System Level)/RConn1 -- Electrical Reference1/LConn1 -- Voltage Sensor/RConn2 -- Battery model/RConn1
  SOC calculation/RConn1 -- Motor & Drive (System Level)/LConn1
  Motor & Drive (System Level)/LConn2 -- Simulink-PS Converter1/RConn1
  Mechanical Rotational Reference/LConn1 -- Motor & Drive (System Level)/RConn4
  Motor & Drive (System Level)/LConn3 -- Speed Sensor/LConn1 -- Motor Reducer/LConn1
  PS Terminator/LConn1 -- Motor & Drive (System Level)/RConn2
  Motor & Drive (System Level)/RConn3 -- Perfect Insulator/LConn1
  SOC calculation/LConn1 -- Voltage Sensor/LConn1 -- Battery model/LConn1
  Battery model/RConn2 -- Temperature Sensor/LConn1
  PS-Simulink Converter1/LConn1 -- Temperature Sensor/RConn1
  PS-Simulink Converter2/LConn1 -- Voltage Sensor/RConn1
  Motor Reducer/RConn1 -- MotorShaftOut/RConn1

== system Tractor_KRAKER_etrailer_v2_2023a_backup050824/Tractor_semitrailer /Kraker etrailer/Etrailer-Controller ==
  RefVehSpeed : Inport
  Vx : Inport  Port=2
  throttle : Inport  Port=3
  brake : Inport  Port=4
  Mb_trailer : Inport  Port=5
  SOC : Inport  Port=6
  Control : Subsystem
      settings: PortSchema="{\"entries\":[{\"content\":{\"sides\":[{\"content\":{\"connectorIds\":[\"Out1\",\"Out2\"]},\"type\":\"ConnectorPlacement.EquallySpacedRectSide\",\"uuid\":\"12b9f2c9-2b28-451b-ad36-7fe4150db485\"},{\"content\":{\"connectorIds\":[\"In1\",\"In2\",\"In3\",\"In4\",\"In5\",\"In6\"],\"side\":\"RIGHT\"},\"type\":\"ConnectorPlacement.EquallySpacedRectSide\",\"uuid\":\"c0fdf9a4-483a-4ddc-b663-6299fcc79327\"},{\"content\":{\"side\":\"TOP\"},\"type\":\"ConnectorPlacement.EquallySpacedRectSide\",\"uuid\":\"3f20082e-8487-45e3-9fd7-d6d75741df4d\"}]},\"type\":\"ConnectorPlacement.EquallySpacedConnector\",\"uuid\":\"9361cdd3-74d8-46ee-ae7f-e2dde5d31ed1\"}],\"packageUris\":[\"http://schema.mathworks.com/mf0/Connector/R2020b\"],\"version\":\"1.0\"}"
  To Workspace : ToWorkspace  VariableName=p_Etrailercontrol_Mb  SampleTime=sp_t
  To Workspace1 : ToWorkspace  VariableName=p_Etrailercontrol_TrqCmd  SampleTime=sp_t
  Mb : Outport
  MotorCmdTrq : Outport  Port=2
  wires:
  RefVehSpeed/1 -> Control/2(SpdRef)
  Control/1(Mbrake) -> To Workspace/1, Mb/1  "Mbrake"
  Control/2(TrqCmd) -> MotorCmdTrq/1, To Workspace1/1  "MotCmdTrq"
  Vx/1 -> Control/1(Vx)
  throttle/1 -> Control/3(throttle)
  brake/1 -> Control/4(brake)
  Mb_trailer/1 -> Control/5(Mb_trailer)
  SOC/1 -> Control/6(SOC)
